simulink model "SW_8"  (R2013b)
settings: Solver=ode45  StartTime=0.0  StopTime=128  RelTol=1e-3
values from neighbouring files (symbols this model uses):
  const_val_lenqs = Nq-1    [confSim.m]    (also in preS_confSim.m)
  g = 1    [confSim.m]
  MiS = -5    [confSim.m]
  MS = 5    [confSim.m]
  nb_counter = ceil(log2(Ns))    [confSim.m]    (also in preS_confSim.m)
  NBitsScoreBus = 10    [confSim.m]    (also in preS_confSim.m)
  Nq = length(qCode)    [confSim.m]    (also in preS_confSim.m)
  Ns = length(sCode)    [confSim.m]    (also in preS_confSim.m)
  qCode = base2dec(q,Base)    [confSim.m]
  sCode = base2dec(s,Base)    [confSim.m]
  SMR_len = Nq*3    [confSim.m]    (also in preS_confSim.m)
libraries: xbsIndex_r4 x1212
(part 1 of 7)
settings Model: Creator=Fabio  LastModifiedBy=fabio

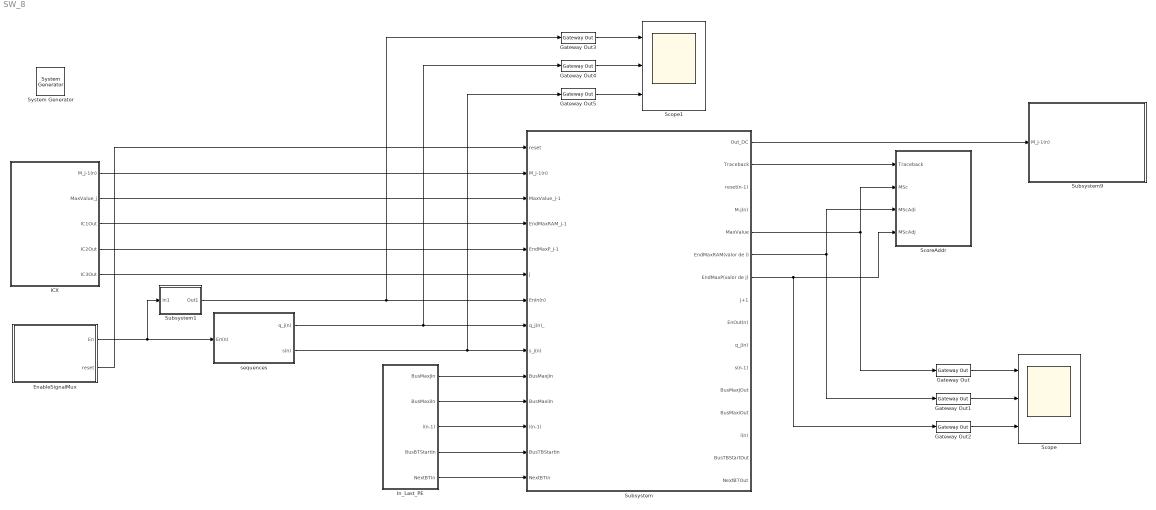
== system SW_8 ==
  " System Generator" : xbsIndex_r4/ System Generator  Tag=genX  xilinxfamily=virtex6  part=xc6vlx240t  speed=-1  package=ff1156  synthesis_tool=XST  clock_wrapper=Clock Enables  directory=./netlist  proj_type=Project Navigator  Synth_file=XST Defaults  Impl_file=ISE Defaults  testbench=off  simulink_period=Ts  sysclk_period=20  dcm_input_clock_period=10  incr_netlist=off  trim_vbits=Everywhere in SubSystem  dbl_ovrd=According to Block Masks  core_generation=According to Block Masks  run_coregen=off  deprecated_control=off  eval_field=0  block_type=sysgen
  "EnableSignalMux " : Subsystem
  Gateway Out{,1..5} (6 alike) : xbsIndex_r4/Gateway Out  inherit_from_input=off  hdl_port=on  timing_constraint=None  locs_specified=off  LOCs={}  UseAsDAC=off  DACChannel='1'  block_type=gatewayout
  ICX : Subsystem
  In_Last_PE : Subsystem
  Scope : Scope  NumInputPorts=3
      settings: YMin=-5~-5~-5  YMax=5~5~5
  Scope1 : Scope  NumInputPorts=3
      settings: YMin=-5~-5~-5  YMax=5~5~5
  ScoreAddr : Subsystem
  Subsystem : Subsystem
  Subsystem1 : Subsystem
  Subsystem9 : Subsystem
  sequences : Subsystem
  wires:
  ICX/1("M_j-1(n) ") -> Subsystem/2(M_j-1(n))
  ICX/2(MaxValue_j) -> Subsystem/3(MaxValue_j-1)
  ICX/3(IC1Out) -> Subsystem/4(EndMaxRAM_j-1)
  ICX/4(IC2Out) -> Subsystem/5(EndMaxP_j-1)
  ICX/5(IC3Out) -> Subsystem/6(j)
  "EnableSignalMux "/2(reset) -> Subsystem/1("reset ")
  In_Last_PE/1(BusMaxjIn) -> Subsystem/10(BusMaxjIn)
  In_Last_PE/2(BusMaxiIn) -> Subsystem/11(BusMaxiIn)
  In_Last_PE/3(i(n-1)) -> Subsystem/12(i(n-1))
  In_Last_PE/4(" BusBTStartIn") -> Subsystem/13(BusTBStartIn)
  In_Last_PE/5(NextBTIn) -> Subsystem/14(NextBTIn)
  Subsystem/1(Out_DC) -> Subsystem9/1(M_j-1(n))
  Subsystem/2(Traceback) -> ScoreAddr/1(Traceback)
  Subsystem/5(MaxValue) -> Gateway Out/1, ScoreAddr/2("MSc ")
  Subsystem/6(EndMaxRAM(valor de i)) -> Gateway Out1/1, ScoreAddr/3(MScAdi)
  Gateway Out/1 -> Scope/1
  Gateway Out1/1 -> Scope/2
  Gateway Out2/1 -> Scope/3
  Subsystem/7(EndMaxP(valor de j)) -> Gateway Out2/1, ScoreAddr/4(MScAdj)
  "EnableSignalMux "/1(En) -> Subsystem1/1(In1), sequences/1(En(n))
  sequences/1(q_j(n)) -> Subsystem/8(q_j(n)_), Gateway Out4/1
  Gateway Out3/1 -> Scope1/1
  Gateway Out4/1 -> Scope1/2
  Gateway Out5/1 -> Scope1/3
  sequences/2(s(n)) -> Gateway Out5/1, Subsystem/9(s_j(n))
  Subsystem1/1(Out1) -> Gateway Out3/1, Subsystem/7(EnIn(n))

== system SW_8/EnableSignalMux  ==
  Accumulator : xbsIndex_r4/Accumulator  operation=Add  n_bits=nbCR  overflow=Saturate  scale=1  rst=on  hasbypass=off  en=on  dbl_ovrd=off  use_behavioral_HDL=on  implementation=Fabric  block_type=accum
  Constant : xbsIndex_r4/Constant  const=1  gui_display_data_type=Fixed-point  arith_type=Unsigned  n_bits=1  bin_pt=0  preci_type=Single  exp_width=8  frac_width=24  explicit_period=on  period=tm  equ=P=C  opselect=C  inp2=PCIN>>17  opr=+  inp1=P  carry=CIN  dbl_ovrd=off  block_type=constant
  Constant1 : xbsIndex_r4/Constant  const=0  gui_display_data_type=Fixed-point  arith_type=Unsigned  n_bits=1  bin_pt=0  preci_type=Single  exp_width=8  frac_width=24  explicit_period=on  period=tm  equ=P=C  opselect=C  inp2=PCIN>>17  opr=+  inp1=P  carry=CIN  dbl_ovrd=off  block_type=constant
  Constant2 : xbsIndex_r4/Constant  const=Ns  gui_display_data_type=Fixed-point  arith_type=Unsigned  n_bits=nb_counter+1  bin_pt=0  preci_type=Single  exp_width=8  frac_width=24  explicit_period=on  period=tm  equ=P=C  opselect=C  inp2=PCIN>>17  opr=+  inp1=P  carry=CIN  dbl_ovrd=off  block_type=constant
  Convert2 : xbsIndex_r4/Convert  gui_display_data_type=Fixed-point  arith_type=Unsigned  n_bits=k  bin_pt=0  float_type=Single  exp_bits=8  fraction_bits=24  quantization=Truncate  overflow=Wrap  en=off  latency=c0  dbl_ovrd=off  pipeline=off  block_type=convert
  Convert5 : xbsIndex_r4/Convert  gui_display_data_type=Boolean  arith_type=Boolean  n_bits=4  bin_pt=0  float_type=Single  exp_bits=8  fraction_bits=24  quantization=Truncate  overflow=Wrap  en=off  latency=c0  dbl_ovrd=off  pipeline=off  block_type=convert
  From Register : xbsIndex_r4/From Register  shared_memory_name='En'  init=1  period=Ts  ownership=Locally owned and initialized  gui_display_data_type=Fixed-point  arith_type=Unsigned  n_bits=2  bin_pt=0  preci_type=Single  dbl_ovrd=off  block_type=fromreg
      settings: AttributesFormatString=<< %<shared_memory_name> >>  infoedit="Register block that reads data to a shared memory register.  Delay of one sample period."
  Inverter : xbsIndex_r4/Inverter  en=off  latency=l0  dbl_ovrd=off  block_type=inv
  Logical : xbsIndex_r4/Logical  logical_function=AND  inputs=2  en=off  latency=0  precision=Full  arith_type=Unsigned  n_bits=16  bin_pt=0  align_bp=on  dbl_ovrd=off  block_type=logical
  Mux : xbsIndex_r4/Mux  inputs=2  en=off  latency=0  precision=User Defined  arith_type=Unsigned  n_bits=nbEnMux  bin_pt=bpEnMux  quantization=Truncate  overflow=Wrap  dbl_ovrd=off  block_type=mux
  Relational : xbsIndex_r4/Relational  mode=a>=b  en=off  latency=r0  dbl_ovrd=off  block_type=relational
  Relational1 : xbsIndex_r4/Relational  mode=a>b  en=off  latency=r0  dbl_ovrd=off  block_type=relational
  "delay_reset " : xbsIndex_r4/Register  init=0  rst=off  en=off  dbl_ovrd=off  block_type=register
  En : Outport
  reset : Outport  Port=2
  wires:
  Constant/1 -> Mux/2
  Constant1/1 -> Relational1/2, Mux/3
  Constant2/1 -> Relational/2
  Accumulator/1 -> Relational/1
  Relational/1 -> Mux/1
  Mux/1 -> Convert5/1
  Convert5/1 -> Logical/2
  Logical/1 -> En/1
  Convert2/1 -> Accumulator/1
  From Register/1 -> Relational1/1
  Inverter/1 -> "delay_reset "/1, Accumulator/2
  "delay_reset "/1 -> reset/1
  Relational1/1 -> Accumulator/3, Logical/1, Convert2/1, Inverter/1

== system SW_8/ICX ==
  "ICM_j-1(n) " : xbsIndex_r4/Constant  const=0  gui_display_data_type=Fixed-point  arith_type=Signed (2's comp)  n_bits=NBitsIn  bin_pt=0  preci_type=Single  exp_width=8  frac_width=24  explicit_period=on  period=t0  equ=P=C  opselect=C  inp2=PCIN>>17  opr=+  inp1=P  carry=CIN  dbl_ovrd=off  block_type=constant
  ICMaxValue__j-1 : xbsIndex_r4/Constant  const=0  gui_display_data_type=Fixed-point  arith_type=Signed (2's comp)  n_bits=NBitsIn  bin_pt=0  preci_type=Single  exp_width=8  frac_width=24  explicit_period=on  period=t0  equ=P=C  opselect=C  inp2=PCIN>>17  opr=+  inp1=P  carry=CIN  dbl_ovrd=off  block_type=constant
  ICOut1 : xbsIndex_r4/Constant  const=0  gui_display_data_type=Fixed-point  arith_type=Signed (2's comp)  n_bits=NBitsIn  bin_pt=0  preci_type=Single  exp_width=8  frac_width=24  explicit_period=on  period=t0  equ=P=C  opselect=C  inp2=PCIN>>17  opr=+  inp1=P  carry=CIN  dbl_ovrd=off  block_type=constant
  ICOut2 : xbsIndex_r4/Constant  const=0  gui_display_data_type=Fixed-point  arith_type=Signed (2's comp)  n_bits=NBitsIn  bin_pt=0  preci_type=Single  exp_width=8  frac_width=24  explicit_period=on  period=t0  equ=P=C  opselect=C  inp2=PCIN>>17  opr=+  inp1=P  carry=CIN  dbl_ovrd=off  block_type=constant
  ICOut3 : xbsIndex_r4/Constant  const=0  gui_display_data_type=Fixed-point  arith_type=Signed (2's comp)  n_bits=NBitsIn  bin_pt=0  preci_type=Single  exp_width=8  frac_width=24  explicit_period=on  period=t0  equ=P=C  opselect=C  inp2=PCIN>>17  opr=+  inp1=P  carry=CIN  dbl_ovrd=off  block_type=constant
  "M_j-1(n) " : Outport
  MaxValue_j : Outport  Port=2
  IC1Out : Outport  Port=3
  IC2Out : Outport  Port=4
  IC3Out : Outport  Port=5
  wires:
  ICMaxValue__j-1/1 -> MaxValue_j/1
  "ICM_j-1(n) "/1 -> "M_j-1(n) "/1
  ICOut3/1 -> IC3Out/1
  ICOut2/1 -> IC2Out/1
  ICOut1/1 -> IC1Out/1

== system SW_8/In_Last_PE ==
  IC : xbsIndex_r4/Constant  const=0  gui_display_data_type=Fixed-point  arith_type=Unsigned  n_bits=3  bin_pt=0  preci_type=Single  exp_width=8  frac_width=24  explicit_period=on  period=Ts  equ=P=C  opselect=C  inp2=PCIN>>17  opr=+  inp1=P  carry=CIN  dbl_ovrd=off  block_type=constant
  IC1 : xbsIndex_r4/Constant  const=0  gui_display_data_type=Fixed-point  arith_type=Unsigned  n_bits=3  bin_pt=0  preci_type=Single  exp_width=8  frac_width=24  explicit_period=on  period=Ts  equ=P=C  opselect=C  inp2=PCIN>>17  opr=+  inp1=P  carry=CIN  dbl_ovrd=off  block_type=constant
  IC2 : xbsIndex_r4/Constant  const=0  gui_display_data_type=Fixed-point  arith_type=Unsigned  n_bits=NBitsIn  bin_pt=0  preci_type=Single  exp_width=8  frac_width=24  explicit_period=on  period=Ts  equ=P=C  opselect=C  inp2=PCIN>>17  opr=+  inp1=P  carry=CIN  dbl_ovrd=off  block_type=constant
  IC3 : xbsIndex_r4/Constant  const=0  gui_display_data_type=Fixed-point  arith_type=Unsigned  n_bits=1  bin_pt=0  preci_type=Single  exp_width=8  frac_width=24  explicit_period=on  period=Ts  equ=P=C  opselect=C  inp2=PCIN>>17  opr=+  inp1=P  carry=CIN  dbl_ovrd=off  block_type=constant
  IC5 : xbsIndex_r4/Constant  const=0  gui_display_data_type=Fixed-point  arith_type=Unsigned  n_bits=1  bin_pt=0  preci_type=Single  exp_width=8  frac_width=24  explicit_period=on  period=Ts  equ=P=C  opselect=C  inp2=PCIN>>17  opr=+  inp1=P  carry=CIN  dbl_ovrd=off  block_type=constant
  BusMaxjIn : Outport
  BusMaxiIn : Outport  Port=2
  i(n-1) : Outport  Port=3
  " BusBTStartIn" : Outport  Port=4
  NextBTIn : Outport  Port=5
  wires:
  IC3/1 -> " BusBTStartIn"/1
  IC1/1 -> BusMaxiIn/1
  IC5/1 -> NextBTIn/1
  IC2/1 -> i(n-1)/1
  IC/1 -> BusMaxjIn/1

== system SW_8/ScoreAddr ==
  Traceback : Inport
  "MSc " : Inport  Port=2
  MScAdi : Inport  Port=3
  MScAdj : Inport  Port=4
  Const_2 : xbsIndex_r4/Constant  const=2  gui_display_data_type=Fixed-point  arith_type=Unsigned  n_bits=k  bin_pt=kbp  preci_type=Single  exp_width=8  frac_width=24  explicit_period=off  period=1  equ=P=C  opselect=C  inp2=PCIN>>17  opr=+  inp1=P  carry=CIN  dbl_ovrd=off  block_type=constant
  Convert1 : xbsIndex_r4/Convert  gui_display_data_type=Boolean  arith_type=Boolean  n_bits=1  bin_pt=0  float_type=Single  exp_bits=8  fraction_bits=24  quantization=Truncate  overflow=Wrap  en=off  latency=c0  dbl_ovrd=off  pipeline=off  block_type=convert
  Counter : xbsIndex_r4/Counter  cnt_type=Count Limited  cnt_to=2  operation=Up  start_count=0  cnt_by_val=1  arith_type=Unsigned  n_bits=2  bin_pt=0  load_pin=off  rst=off  en=on  explicit_period=on  period=Ts  dbl_ovrd=off  use_behavioral_HDL=off  implementation=Fabric  block_type=counter
  Mux3 : xbsIndex_r4/Mux  inputs=3  en=off  latency=mft  precision=User Defined  arith_type=Unsigned  n_bits=NBitsCalcInt  bin_pt=0  quantization=Truncate  overflow=Wrap  dbl_ovrd=off  block_type=mux
  Register1 : xbsIndex_r4/Register  init=0  rst=on  en=on  dbl_ovrd=off  block_type=register
  Relational : xbsIndex_r4/Relational  mode=a=b  en=off  latency=0  dbl_ovrd=off  block_type=relational
  Shared Memory : xbsIndex_r4/Shared Memory  shared_memory_name='ScrnAddrs'  depth=3  ownership=Locally Owned and Initialized  initVector=zeros(1,3)  en=off  mutex=Unprotected  mode=Write Only  write_mode=No Read On Write  time_out=0  latency=Ts  explicit_data_type=on  gui_display_data_type=Fixed-point  arith_type=Unsigned  n_bits=16  bin_pt=0  preci_type=Single  implementation=Block RAM  use_rpm=off  block_type=shmem
      settings: AttributesFormatString=<< %<shared_memory_name> >>
  setEnable : Subsystem
  wires:
  Const_2/1 -> Relational/1
  Convert1/1 -> setEnable/1(In1), Register1/3, Register1/1
  Register1/1 -> Shared Memory/3
  Mux3/1 -> Shared Memory/2
  Counter/1 -> Relational/2, Shared Memory/1, Mux3/1
  "MSc "/1 -> Mux3/2
  MScAdi/1 -> Mux3/3
  setEnable/1(Out1) -> Counter/1
  Relational/1 -> Register1/2
  MScAdj/1 -> Mux3/4
  Traceback/1 -> Convert1/1

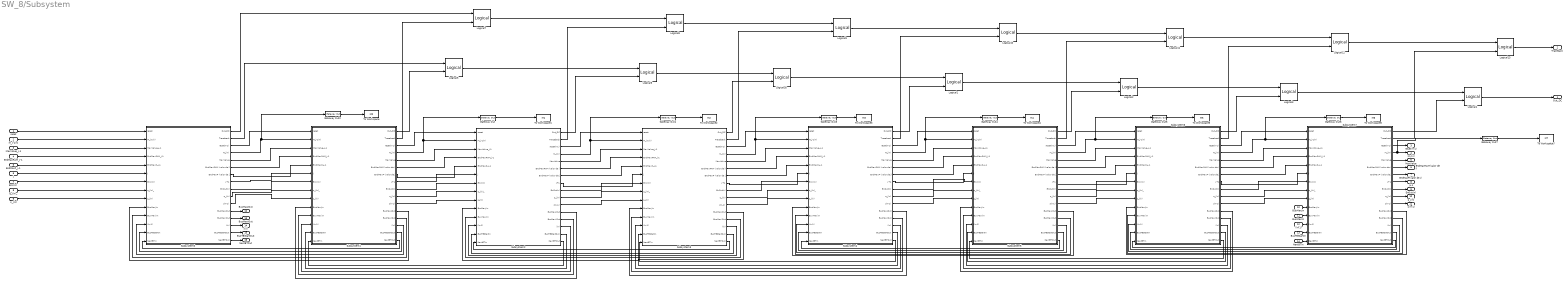
== system SW_8/Subsystem ==
  "reset " : Inport
  M_j-1(n) : Inport  Port=2
  MaxValue_j-1 : Inport  Port=3
  EndMaxRAM_j-1 : Inport  Port=4
  EndMaxP_j-1 : Inport  Port=5
  j : Inport  Port=6
  EnIn(n) : Inport  Port=7
  q_j(n)_ : Inport  Port=8
  s_j(n) : Inport  Port=9
  BusMaxjIn : Inport  Port=10
  BusMaxiIn : Inport  Port=11
  i(n-1) : Inport  Port=12
  BusTBStartIn : Inport  Port=13
  NextBTIn : Inport  Port=14
  Gateway Out{,1..7} (8 alike) : xbsIndex_r4/Gateway Out  inherit_from_input=off  hdl_port=on  timing_constraint=None  locs_specified=off  LOCs={}  UseAsDAC=off  DACChannel='1'  block_type=gatewayout
  Logical{1..6,35} (7 alike) : xbsIndex_r4/Logical  logical_function=XOR  inputs=2  en=off  latency=l0  precision=User Defined  arith_type=Unsigned  n_bits=k  bin_pt=0  align_bp=on  dbl_ovrd=off  block_type=logical
  Logical{7..13} (7 alike) : xbsIndex_r4/Logical  logical_function=XOR  inputs=2  en=off  latency=l0  precision=User Defined  arith_type=Unsigned  n_bits=nb_bool  bin_pt=0  align_bp=on  dbl_ovrd=off  block_type=logical
  Subsystem0 : Subsystem
  Subsystem1 : Subsystem
  Subsystem2 : Subsystem
  Subsystem3 : Subsystem
  Subsystem4 : Subsystem
  Subsystem5 : Subsystem
  Subsystem6 : Subsystem
  Subsystem7 : Subsystem
  To Workspace : ToWorkspace  VariableName=M0  SampleTime=-1
  To Workspace1 : ToWorkspace  VariableName=M1  SampleTime=-1
  To Workspace2 : ToWorkspace  VariableName=M2  SampleTime=-1
  To Workspace3 : ToWorkspace  VariableName=M3  SampleTime=-1
  To Workspace4 : ToWorkspace  VariableName=M4  SampleTime=-1
  To Workspace5 : ToWorkspace  VariableName=M5  SampleTime=-1
  To Workspace6 : ToWorkspace  VariableName=M6  SampleTime=-1
  To Workspace7 : ToWorkspace  VariableName=M7  SampleTime=-1
  Out_DC : Outport
  Traceback : Outport  Port=2
  reset(n-1) : Outport  Port=3
  M-j(n) : Outport  Port=4
  MaxValue : Outport  Port=5
  EndMaxRAM(valor de i) : Outport  Port=6
  EndMaxP(valor de j) : Outport  Port=7
  j+1 : Outport  Port=8
  EnOut(n) : Outport  Port=9
  q_j(n) : Outport  Port=10
  s(n-1) : Outport  Port=11
  BusMaxjOut : Outport  Port=12
  BusMaxiOut : Outport  Port=13
  i(n) : Outport  Port=14
  BusTBStartOut : Outport  Port=15
  NextBTOut : Outport  Port=16
  wires:
  Subsystem4/1("Out_DC ") -> Logical1/2
  s_j(n)/1 -> Subsystem0/9(s_j(n))
  M_j-1(n)/1 -> Subsystem0/2(M_j-1(n))
  j/1 -> Subsystem0/6(j)
  EndMaxRAM_j-1/1 -> Subsystem0/4(EndMaxRAM_j-1)
  MaxValue_j-1/1 -> Subsystem0/3(MaxValue_j-1)
  q_j(n)_/1 -> Subsystem0/8(q_j(n)_)
  EndMaxP_j-1/1 -> Subsystem0/5(EndMaxP_j-1)
  EnIn(n)/1 -> Subsystem0/7(EnIn(n))
  BusTBStartIn/1 -> Subsystem7/13(BusTBStartIn)
  NextBTIn/1 -> Subsystem7/14(NextBTIn)
  Subsystem7/5(MaxValue) -> MaxValue/1
  Subsystem7/6(EndMaxRAM (valor de i)) -> EndMaxRAM(valor de i)/1
  Subsystem7/7(EndMaxP (valor de j)) -> EndMaxP(valor de j)/1
  Subsystem7/8(j+1) -> j+1/1
  Subsystem7/9(EnOut(n)) -> EnOut(n)/1
  Subsystem7/10(q_j(n)) -> q_j(n)/1
  Subsystem7/11(s(n-1)) -> s(n-1)/1
  Logical35/1 -> Logical1/1
  Logical1/1 -> Logical2/1
  Subsystem3/1("Out_DC ") -> Logical35/2
  Subsystem7/1("Out_DC ") -> Logical4/2
  Logical2/1 -> Logical3/1
  Logical3/1 -> Logical4/1
  Subsystem6/1("Out_DC ") -> Logical3/2
  Subsystem5/2(Traceback) -> Logical11/2
  Subsystem5/1("Out_DC ") -> Logical2/2
  Logical9/1 -> Logical10/1
  Logical4/1 -> Out_DC/1
  Subsystem0/12(BusMaxjOut) -> BusMaxjOut/1
  Logical13/1 -> Traceback/1
  Subsystem0/13(BusMaxiOut) -> BusMaxiOut/1
  Subsystem0/16(NextBTOut) -> NextBTOut/1
  BusMaxiIn/1 -> Subsystem7/11(BuxMaxiIn)
  i(n-1)/1 -> Subsystem7/12(i(n-1))
  Subsystem0/15(BusTBStartOut) -> BusTBStartOut/1
  BusMaxjIn/1 -> Subsystem7/10(BusMaxjIn)
  Subsystem0/14(i(n)) -> i(n)/1
  Subsystem1/1("Out_DC ") -> Logical5/2
  Logical12/1 -> Logical13/1
  Subsystem2/2(Traceback) -> Logical8/2
  Logical7/1 -> Logical8/1
  Subsystem7/2(Traceback) -> Logical13/2
  Logical11/1 -> Logical12/1
  Logical8/1 -> Logical9/1
  Logical10/1 -> Logical11/1
  Logical6/1 -> Logical35/1
  Subsystem6/2(Traceback) -> Logical12/2
  Subsystem3/2(Traceback) -> Logical9/2
  Logical5/1 -> Logical6/1
  Subsystem2/1("Out_DC ") -> Logical6/2
  Subsystem4/2(Traceback) -> Logical10/2
  "reset "/1 -> Subsystem0/1("reset ")
  Subsystem0/3(reset(n-1)) -> Subsystem1/1("reset ")
  Subsystem0/5(MaxValue) -> Subsystem1/3(MaxValue_j-1)
  Subsystem0/6(EndMaxRAM (valor de i)) -> Subsystem1/4(EndMaxRAM_j-1)
  Subsystem0/7(EndMaxP (valor de j)) -> Subsystem1/5(EndMaxP_j-1)
  Subsystem0/8(j+1) -> Subsystem1/6(j)
  Subsystem0/9(EnOut(n)) -> Subsystem1/7(EnIn(n))
  Subsystem0/10(q_j(n)) -> Subsystem1/8(q_j(n)_)
  Subsystem0/11(s(n-1)) -> Subsystem1/9(s_j(n))
  Subsystem1/3(reset(n-1)) -> Subsystem2/1("reset ")
  Subsystem1/5(MaxValue) -> Subsystem2/3(MaxValue_j-1)
  Subsystem1/6(EndMaxRAM (valor de i)) -> Subsystem2/4(EndMaxRAM_j-1)
  Subsystem1/7(EndMaxP (valor de j)) -> Subsystem2/5(EndMaxP_j-1)
  Subsystem1/8(j+1) -> Subsystem2/6(j)
  Subsystem1/9(EnOut(n)) -> Subsystem2/7(EnIn(n))
  Subsystem1/10(q_j(n)) -> Subsystem2/8(q_j(n)_)
  Subsystem1/11(s(n-1)) -> Subsystem2/9(s_j(n))
  Subsystem2/3(reset(n-1)) -> Subsystem3/1("reset ")
  Subsystem2/5(MaxValue) -> Subsystem3/3(MaxValue_j-1)
  Subsystem2/6(EndMaxRAM (valor de i)) -> Subsystem3/4(EndMaxRAM_j-1)
  Subsystem2/7(EndMaxP (valor de j)) -> Subsystem3/5(EndMaxP_j-1)
  Subsystem2/8(j+1) -> Subsystem3/6(j)
  Subsystem2/9(EnOut(n)) -> Subsystem3/7(EnIn(n))
  Subsystem2/10(q_j(n)) -> Subsystem3/8(q_j(n)_)
  Subsystem2/11(s(n-1)) -> Subsystem3/9(s_j(n))
  Subsystem3/3(reset(n-1)) -> Subsystem4/1("reset ")
  Subsystem3/5(MaxValue) -> Subsystem4/3(MaxValue_j-1)
  Subsystem3/6(EndMaxRAM (valor de i)) -> Subsystem4/4(EndMaxRAM_j-1)
  Subsystem3/7(EndMaxP (valor de j)) -> Subsystem4/5(EndMaxP_j-1)
  Subsystem3/8(j+1) -> Subsystem4/6(j)
  Subsystem3/9(EnOut(n)) -> Subsystem4/7(EnIn(n))
  Subsystem3/10(q_j(n)) -> Subsystem4/8(q_j(n)_)
  Subsystem3/11(s(n-1)) -> Subsystem4/9(s_j(n))
  Subsystem4/3(reset(n-1)) -> Subsystem5/1("reset ")
  Subsystem4/5(MaxValue) -> Subsystem5/3(MaxValue_j-1)
  Subsystem4/6(EndMaxRAM (valor de i)) -> Subsystem5/4(EndMaxRAM_j-1)
  Subsystem4/7(EndMaxP (valor de j)) -> Subsystem5/5(EndMaxP_j-1)
  Subsystem4/8(j+1) -> Subsystem5/6(j)
  Subsystem4/9(EnOut(n)) -> Subsystem5/7(EnIn(n))
  Subsystem4/10(q_j(n)) -> Subsystem5/8(q_j(n)_)
  Subsystem4/11(s(n-1)) -> Subsystem5/9(s_j(n))
  Subsystem5/3(reset(n-1)) -> Subsystem6/1("reset ")
  Subsystem5/5(MaxValue) -> Subsystem6/3(MaxValue_j-1)
  Subsystem5/6(EndMaxRAM (valor de i)) -> Subsystem6/4(EndMaxRAM_j-1)
  Subsystem5/7(EndMaxP (valor de j)) -> Subsystem6/5(EndMaxP_j-1)
  Subsystem5/8(j+1) -> Subsystem6/6(j)
  Subsystem5/9(EnOut(n)) -> Subsystem6/7(EnIn(n))
  Subsystem5/10(q_j(n)) -> Subsystem6/8(q_j(n)_)
  Subsystem5/11(s(n-1)) -> Subsystem6/9(s_j(n))
  Subsystem6/3(reset(n-1)) -> Subsystem7/1("reset ")
  Subsystem6/5(MaxValue) -> Subsystem7/3(MaxValue_j-1)
  Subsystem6/6(EndMaxRAM (valor de i)) -> Subsystem7/4(EndMaxRAM_j-1)
  Subsystem6/7(EndMaxP (valor de j)) -> Subsystem7/5(EndMaxP_j-1)
  Subsystem6/8(j+1) -> Subsystem7/6(j)
  Subsystem6/9(EnOut(n)) -> Subsystem7/7(EnIn(n))
  Subsystem6/10(q_j(n)) -> Subsystem7/8(q_j(n)_)
  Subsystem6/11(s(n-1)) -> Subsystem7/9(s_j(n))
  Subsystem7/3(reset(n-1)) -> reset(n-1)/1
  Subsystem1/2(Traceback) -> Logical7/2
  Subsystem7/16(NextBTOut) -> Subsystem6/14(NextBTIn)
  Subsystem7/15(BusTBStartOut) -> Subsystem6/13(BusTBStartIn)
  Subsystem7/14(i(n)) -> Subsystem6/12(i(n-1))
  Subsystem3/16(NextBTOut) -> Subsystem2/14(NextBTIn)
  Subsystem7/13(BusMaxiOut) -> Subsystem6/11(BuxMaxiIn)
  Subsystem7/12(BusMaxjOut) -> Subsystem6/10(BusMaxjIn)
  Subsystem6/16(NextBTOut) -> Subsystem5/14(NextBTIn)
  Subsystem6/15(BusTBStartOut) -> Subsystem5/13(BusTBStartIn)
  Subsystem6/14(i(n)) -> Subsystem5/12(i(n-1))
  Subsystem6/13(BusMaxiOut) -> Subsystem5/11(BuxMaxiIn)
  Subsystem6/12(BusMaxjOut) -> Subsystem5/10(BusMaxjIn)
  Subsystem5/16(NextBTOut) -> Subsystem4/14(NextBTIn)
  Subsystem5/15(BusTBStartOut) -> Subsystem4/13(BusTBStartIn)
  Subsystem5/14(i(n)) -> Subsystem4/12(i(n-1))
  Subsystem5/13(BusMaxiOut) -> Subsystem4/11(BuxMaxiIn)
  Subsystem5/12(BusMaxjOut) -> Subsystem4/10(BusMaxjIn)
  Subsystem4/16(NextBTOut) -> Subsystem3/14(NextBTIn)
  Subsystem4/15(BusTBStartOut) -> Subsystem3/13(BusTBStartIn)
  Subsystem4/14(i(n)) -> Subsystem3/12(i(n-1))
  Subsystem4/13(BusMaxiOut) -> Subsystem3/11(BuxMaxiIn)
  Subsystem4/12(BusMaxjOut) -> Subsystem3/10(BusMaxjIn)
  Subsystem3/15(BusTBStartOut) -> Subsystem2/13(BusTBStartIn)
  Subsystem3/14(i(n)) -> Subsystem2/12(i(n-1))
  Subsystem3/13(BusMaxiOut) -> Subsystem2/11(BuxMaxiIn)
  Subsystem3/12(BusMaxjOut) -> Subsystem2/10(BusMaxjIn)
  Subsystem2/16(NextBTOut) -> Subsystem1/14(NextBTIn)
  Subsystem2/15(BusTBStartOut) -> Subsystem1/13(BusTBStartIn)
  Subsystem2/14(i(n)) -> Subsystem1/12(i(n-1))
  Subsystem2/13(BusMaxiOut) -> Subsystem1/11(BuxMaxiIn)
  Subsystem2/12(BusMaxjOut) -> Subsystem1/10(BusMaxjIn)
  Subsystem1/16(NextBTOut) -> Subsystem0/14(NextBTIn)
  Subsystem1/15(BusTBStartOut) -> Subsystem0/13(BusTBStartIn)
  Subsystem1/14(i(n)) -> Subsystem0/12(i(n-1))
  Subsystem1/13(BusMaxiOut) -> Subsystem0/11(BuxMaxiIn)
  Subsystem1/12(BusMaxjOut) -> Subsystem0/10(BusMaxjIn)
  Subsystem0/4(M_j(n)) -> Gateway Out2/1, Subsystem1/2(M_j-1(n))
  Subsystem1/4(M_j(n)) -> Gateway Out/1, Subsystem2/2(M_j-1(n))
  Subsystem2/4(M_j(n)) -> Gateway Out1/1, Subsystem3/2(M_j-1(n))
  Subsystem3/4(M_j(n)) -> Gateway Out3/1, Subsystem4/2(M_j-1(n))
  Subsystem4/4(M_j(n)) -> Gateway Out4/1, Subsystem5/2(M_j-1(n))
  Subsystem5/4(M_j(n)) -> Gateway Out5/1, Subsystem6/2(M_j-1(n))
  Subsystem6/4(M_j(n)) -> Gateway Out6/1, Subsystem7/2(M_j-1(n))
  Subsystem7/4(M_j(n)) -> Gateway Out7/1, M-j(n)/1
  Gateway Out/1 -> To Workspace1/1
  Gateway Out1/1 -> To Workspace2/1
  Gateway Out2/1 -> To Workspace/1
  Gateway Out3/1 -> To Workspace3/1
  Gateway Out4/1 -> To Workspace4/1
  Gateway Out5/1 -> To Workspace5/1
  Gateway Out6/1 -> To Workspace6/1
  Gateway Out7/1 -> To Workspace7/1
  Subsystem0/1("Out_DC ") -> Logical7/1
  Subsystem0/2(Traceback) -> Logical5/1

== system SW_8/Subsystem1 ==
  In1 : Inport
  Register1 : xbsIndex_r4/Register  init=0  rst=off  en=off  dbl_ovrd=off  block_type=register
  Register2 : xbsIndex_r4/Register  init=0  rst=off  en=off  dbl_ovrd=off  block_type=register
  Out1 : Outport
  wires:
  In1/1 -> Register2/1
  Register1/1 -> Out1/1
  Register2/1 -> Register1/1

== system SW_8/Subsystem9 ==
  M_j-1(n) : Inport
  Accumulator : xbsIndex_r4/Accumulator  operation=Add  n_bits=nb_SMR  overflow=Saturate  scale=1  rst=off  hasbypass=off  en=off  dbl_ovrd=off  use_behavioral_HDL=on  implementation=Fabric  block_type=accum
  Const_2 : xbsIndex_r4/Constant  const=0  gui_display_data_type=Fixed-point  arith_type=Unsigned  n_bits=counter_num_b  bin_pt=kbp  preci_type=Single  exp_width=8  frac_width=24  explicit_period=off  period=1  equ=P=C  opselect=C  inp2=PCIN>>17  opr=+  inp1=P  carry=CIN  dbl_ovrd=off  block_type=constant
  Convert1 : xbsIndex_r4/Convert  gui_display_data_type=Boolean  arith_type=Boolean  n_bits=1  bin_pt=0  float_type=Single  exp_bits=8  fraction_bits=24  quantization=Truncate  overflow=Wrap  en=off  latency=c0  dbl_ovrd=off  pipeline=off  block_type=convert
  Convert2 : xbsIndex_r4/Convert  gui_display_data_type=Fixed-point  arith_type=Unsigned  n_bits=nb_bool  bin_pt=0  float_type=Single  exp_bits=8  fraction_bits=24  quantization=Truncate  overflow=Wrap  en=off  latency=c0  dbl_ovrd=off  pipeline=off  block_type=convert
  Register : xbsIndex_r4/Register  init=0  rst=off  en=off  dbl_ovrd=off  block_type=register
  Register1 : xbsIndex_r4/Register  init=0  rst=off  en=off  dbl_ovrd=off  block_type=register
  Register2 : xbsIndex_r4/Register  init=0  rst=off  en=off  dbl_ovrd=off  block_type=register
  Relational : xbsIndex_r4/Relational  mode=a<b  en=off  latency=r0  dbl_ovrd=off  block_type=relational
  Shared Memory : xbsIndex_r4/Shared Memory  shared_memory_name='SMR2'  depth=SMR_len  ownership=Locally Owned and Initialized  initVector=zeros(1,SMR_len)  en=off  mutex=Unprotected  mode=Write Only  write_mode=No Read On Write  time_out=0  latency=Ts  explicit_data_type=on  gui_display_data_type=Fixed-point  arith_type=Unsigned  n_bits=k  bin_pt=kbp  preci_type=Single  implementation=Block RAM  use_rpm=off  block_type=shmem
      settings: AttributesFormatString=<< %<shared_memory_name> >>
  wires:
  Register/1 -> Shared Memory/2
  Convert2/1 -> Convert1/1, Accumulator/1
  Relational/1 -> Convert2/1
  Register2/1 -> Shared Memory/1
  Convert1/1 -> Register1/1
  Const_2/1 -> Relational/1
  Accumulator/1 -> Register2/1
  Register1/1 -> Shared Memory/3
  M_j-1(n)/1 -> Relational/2, Register/1

== system SW_8/sequences ==
  En(n) : Inport
  Convert : xbsIndex_r4/Convert  gui_display_data_type=Fixed-point  arith_type=Unsigned  n_bits=nb_bool  bin_pt=bp_bool  float_type=Single  exp_bits=8  fraction_bits=24  quantization=Truncate  overflow=Wrap  en=off  latency=0  dbl_ovrd=off  pipeline=off  block_type=convert
  "qCode " : Subsystem
  sCode : Subsystem
  q_j(n) : Outport
  s(n) : Outport  Port=2
  wires:
  "qCode "/1(qc) -> q_j(n)/1
  sCode/1(sc) -> s(n)/1
  En(n)/1 -> Convert/1
  Convert/1 -> sCode/1(EnS), "qCode "/1("EnQ ")

== system SW_8/ScoreAddr/setEnable ==
  In1 : Inport
  Register1 : xbsIndex_r4/Register  init=0  rst=off  en=on  dbl_ovrd=off  block_type=register
  Out1 : Outport
  wires:
  Register1/1 -> Out1/1
  In1/1 -> Register1/2, Register1/1

== system SW_8/Subsystem/Subsystem0 ==
  "reset " : Inport
  M_j-1(n) : Inport  Port=2
  MaxValue_j-1 : Inport  Port=3
  EndMaxRAM_j-1 : Inport  Port=4
  EndMaxP_j-1 : Inport  Port=5
  j : Inport  Port=6
  EnIn(n) : Inport  Port=7
  q_j(n)_ : Inport  Port=8
  s_j(n) : Inport  Port=9
  BusMaxjIn : Inport  Port=10
  BuxMaxiIn : Inport  Port=11
  i(n-1) : Inport  Port=12
  BusTBStartIn : Inport  Port=13
  NextBTIn : Inport  Port=14
  Backtracking_final : Subsystem
  P1_HW0 : Subsystem
  Register1 : xbsIndex_r4/Register  init=0  rst=off  en=off  dbl_ovrd=off  block_type=register
  Register10 : xbsIndex_r4/Register  init=0  rst=off  en=off  dbl_ovrd=off  block_type=register
  _RAM_0 : Subsystem
  "delay_reset " : xbsIndex_r4/Register  init=0  rst=off  en=off  dbl_ovrd=off  block_type=register
  delay_tc{,1..7} (8 alike) : xbsIndex_r4/Register  init=0  rst=off  en=off  dbl_ovrd=off  block_type=register
  seq_switch : Subsystem
  "Out_DC " : Outport
  Traceback : Outport  Port=2
  reset(n-1) : Outport  Port=3
  M_j(n) : Outport  Port=4
  MaxValue : Outport  Port=5
  EndMaxRAM (valor de i) : Outport  Port=6
  EndMaxP (valor de j) : Outport  Port=7
  j+1 : Outport  Port=8
  EnOut(n) : Outport  Port=9
  q_j(n) : Outport  Port=10
  s(n-1) : Outport  Port=11
  BusMaxjOut : Outport  Port=12
  BusMaxiOut : Outport  Port=13
  i(n) : Outport  Port=14
  BusTBStartOut : Outport  Port=15
  NextBTOut : Outport  Port=16
  wires:
  Backtracking_final/3(Out_DC_j(n)) -> Register10/1
  _RAM_0/1(D_j(n)1) -> Backtracking_final/2("D(j)_n ")
  delay_tc7/1 -> BusMaxjOut/1
  delay_tc6/1 -> NextBTOut/1
  delay_tc5/1 -> i(n)/1
  delay_tc4/1 -> BusTBStartOut/1
  delay_tc3/1 -> BusMaxiOut/1
  delay_tc/1 -> MaxValue/1
  delay_tc2/1 -> EndMaxP (valor de j)/1
  delay_tc1/1 -> EndMaxRAM (valor de i)/1
  EndMaxRAM_j-1/1 -> P1_HW0/4(EndMaxRAM_j-1)
  M_j-1(n)/1 -> P1_HW0/2(M_j-1(n)1)
  j/1 -> P1_HW0/6(j-1)
  seq_switch/1(q_j) -> P1_HW0/9(q_j)
  MaxValue_j-1/1 -> P1_HW0/3(MaxValue_j-1)
  EndMaxP_j-1/1 -> P1_HW0/5(EndMaxP_j-1)
  EnIn(n)/1 -> P1_HW0/8(EnIn), _RAM_0/1(En(n)), seq_switch/2("Enable ")
  Backtracking_final/6(BusTBStartOut) -> delay_tc4/1
  Backtracking_final/8(NextBTOut) -> delay_tc6/1
  BusMaxjIn/1 -> Backtracking_final/7(BusMaxjIn)
  BusTBStartIn/1 -> Backtracking_final/9(BusTBStartIn)
  NextBTIn/1 -> Backtracking_final/11(NextBTIn)
  P1_HW0/11(out_j) -> Backtracking_final/6(j)
  P1_HW0/3(EndMaxRAM (valor de i)) -> Backtracking_final/5(Maxi), delay_tc1/1
  Backtracking_final/1(BT_RAM_j(n)=i) -> _RAM_0/4(BT_RAM_j(n)=i)
  i(n-1)/1 -> Backtracking_final/10(i(n-1))
  Backtracking_final/4(BusMaxjOut) -> delay_tc7/1
  Backtracking_final/5(BusMaxiOut) -> delay_tc3/1
  BuxMaxiIn/1 -> Backtracking_final/8(BusMaxiIn)
  Backtracking_final/7(i(n)) -> delay_tc5/1
  Backtracking_final/2(BTRAMCont) -> _RAM_0/5(BTRAMCont)
  P1_HW0/4(EndMaxP (valor de j)) -> Backtracking_final/4(Maxj), delay_tc2/1
  P1_HW0/1(M_j(n)) -> M_j(n)/1
  P1_HW0/2(MaxValue) -> delay_tc/1
  P1_HW0/9(wEnd) -> _RAM_0/2(RAM_j(n)=i)
  P1_HW0/8(Direction) -> _RAM_0/3(D_j(n))
  P1_HW0/6(s(n-1)) -> s(n-1)/1
  P1_HW0/5(j) -> j+1/1
  P1_HW0/7(EnOut(n)) -> EnOut(n)/1
  seq_switch/2(q_j(n-1)) -> q_j(n)/1
  q_j(n)_/1 -> seq_switch/1(q_j(n))
  s_j(n)/1 -> P1_HW0/7(s(n))
  P1_HW0/10(TraceBackStart) -> Backtracking_final/3(TraceBackStart), Register1/1
  "reset "/1 -> P1_HW0/1("reset "), Backtracking_final/1("reset "), "delay_reset "/1, seq_switch/3("reset ")
  "delay_reset "/1 -> reset(n-1)/1
  Register10/1 -> "Out_DC "/1
  Register1/1 -> Traceback/1

== system SW_8/Subsystem/Subsystem1 ==
  "reset " : Inport
  M_j-1(n) : Inport  Port=2
  MaxValue_j-1 : Inport  Port=3
  EndMaxRAM_j-1 : Inport  Port=4
  EndMaxP_j-1 : Inport  Port=5
  j : Inport  Port=6
  EnIn(n) : Inport  Port=7
  q_j(n)_ : Inport  Port=8
  s_j(n) : Inport  Port=9
  BusMaxjIn : Inport  Port=10
  BuxMaxiIn : Inport  Port=11
  i(n-1) : Inport  Port=12
  BusTBStartIn : Inport  Port=13
  NextBTIn : Inport  Port=14
  Backtracking_final : Subsystem
  P1_HW0 : Subsystem
  Register1 : xbsIndex_r4/Register  init=0  rst=off  en=off  dbl_ovrd=off  block_type=register
  Register10 : xbsIndex_r4/Register  init=0  rst=off  en=off  dbl_ovrd=off  block_type=register
  _RAM_0 : Subsystem
  "delay_reset " : xbsIndex_r4/Register  init=0  rst=off  en=off  dbl_ovrd=off  block_type=register
  delay_tc{,1..7} (8 alike) : xbsIndex_r4/Register  init=0  rst=off  en=off  dbl_ovrd=off  block_type=register
  seq_switch : Subsystem
  "Out_DC " : Outport
  Traceback : Outport  Port=2
  reset(n-1) : Outport  Port=3
  M_j(n) : Outport  Port=4
  MaxValue : Outport  Port=5
  EndMaxRAM (valor de i) : Outport  Port=6
  EndMaxP (valor de j) : Outport  Port=7
  j+1 : Outport  Port=8
  EnOut(n) : Outport  Port=9
  q_j(n) : Outport  Port=10
  s(n-1) : Outport  Port=11
  BusMaxjOut : Outport  Port=12
  BusMaxiOut : Outport  Port=13
  i(n) : Outport  Port=14
  BusTBStartOut : Outport  Port=15
  NextBTOut : Outport  Port=16
  wires:
  Backtracking_final/3(Out_DC_j(n)) -> Register10/1
  _RAM_0/1(D_j(n)1) -> Backtracking_final/2("D(j)_n ")
  delay_tc7/1 -> BusMaxjOut/1
  delay_tc6/1 -> NextBTOut/1
  delay_tc5/1 -> i(n)/1
  delay_tc4/1 -> BusTBStartOut/1
  delay_tc3/1 -> BusMaxiOut/1
  delay_tc/1 -> MaxValue/1
  delay_tc2/1 -> EndMaxP (valor de j)/1
  delay_tc1/1 -> EndMaxRAM (valor de i)/1
  EndMaxRAM_j-1/1 -> P1_HW0/4(EndMaxRAM_j-1)
  M_j-1(n)/1 -> P1_HW0/2(M_j-1(n)1)
  j/1 -> P1_HW0/6(j-1)
  seq_switch/1(q_j) -> P1_HW0/9(q_j)
  MaxValue_j-1/1 -> P1_HW0/3(MaxValue_j-1)
  EndMaxP_j-1/1 -> P1_HW0/5(EndMaxP_j-1)
  EnIn(n)/1 -> P1_HW0/8(EnIn), seq_switch/2("Enable "), _RAM_0/1(En(n))
  Backtracking_final/6(BusTBStartOut) -> delay_tc4/1
  Backtracking_final/8(NextBTOut) -> delay_tc6/1
  BusMaxjIn/1 -> Backtracking_final/7(BusMaxjIn)
  BusTBStartIn/1 -> Backtracking_final/9(BusTBStartIn)
  NextBTIn/1 -> Backtracking_final/11(NextBTIn)
  P1_HW0/11(out_j) -> Backtracking_final/6(j)
  P1_HW0/3(EndMaxRAM (valor de i)) -> Backtracking_final/5(Maxi), delay_tc1/1
  Backtracking_final/1(BT_RAM_j(n)=i) -> _RAM_0/4(BT_RAM_j(n)=i)
  i(n-1)/1 -> Backtracking_final/10(i(n-1))
  Backtracking_final/4(BusMaxjOut) -> delay_tc7/1
  Backtracking_final/5(BusMaxiOut) -> delay_tc3/1
  BuxMaxiIn/1 -> Backtracking_final/8(BusMaxiIn)
  Backtracking_final/7(i(n)) -> delay_tc5/1
  Backtracking_final/2(BTRAMCont) -> _RAM_0/5(BTRAMCont)
  P1_HW0/4(EndMaxP (valor de j)) -> Backtracking_final/4(Maxj), delay_tc2/1
  P1_HW0/1(M_j(n)) -> M_j(n)/1
  P1_HW0/2(MaxValue) -> delay_tc/1
  P1_HW0/9(wEnd) -> _RAM_0/2(RAM_j(n)=i)
  P1_HW0/8(Direction) -> _RAM_0/3(D_j(n))
  P1_HW0/6(s(n-1)) -> s(n-1)/1
  P1_HW0/5(j) -> j+1/1
  P1_HW0/7(EnOut(n)) -> EnOut(n)/1
  seq_switch/2(q_j(n-1)) -> q_j(n)/1
  q_j(n)_/1 -> seq_switch/1(q_j(n))
  s_j(n)/1 -> P1_HW0/7(s(n))
  P1_HW0/10(TraceBackStart) -> Backtracking_final/3(TraceBackStart), Register1/1
  "reset "/1 -> P1_HW0/1("reset "), Backtracking_final/1("reset "), "delay_reset "/1, seq_switch/3("reset ")
  "delay_reset "/1 -> reset(n-1)/1
  Register10/1 -> "Out_DC "/1
  Register1/1 -> Traceback/1

== system SW_8/Subsystem/Subsystem2 ==
  "reset " : Inport
  M_j-1(n) : Inport  Port=2
  MaxValue_j-1 : Inport  Port=3
  EndMaxRAM_j-1 : Inport  Port=4
  EndMaxP_j-1 : Inport  Port=5
  j : Inport  Port=6
  EnIn(n) : Inport  Port=7
  q_j(n)_ : Inport  Port=8
  s_j(n) : Inport  Port=9
  BusMaxjIn : Inport  Port=10
  BuxMaxiIn : Inport  Port=11
  i(n-1) : Inport  Port=12
  BusTBStartIn : Inport  Port=13
  NextBTIn : Inport  Port=14
  Backtracking_final : Subsystem
  P1_HW0 : Subsystem
  Register1 : xbsIndex_r4/Register  init=0  rst=off  en=off  dbl_ovrd=off  block_type=register
  Register10 : xbsIndex_r4/Register  init=0  rst=off  en=off  dbl_ovrd=off  block_type=register
  _RAM_0 : Subsystem
  "delay_reset " : xbsIndex_r4/Register  init=0  rst=off  en=off  dbl_ovrd=off  block_type=register
  delay_tc{,1..7} (8 alike) : xbsIndex_r4/Register  init=0  rst=off  en=off  dbl_ovrd=off  block_type=register
  seq_switch : Subsystem
  "Out_DC " : Outport
  Traceback : Outport  Port=2
  reset(n-1) : Outport  Port=3
  M_j(n) : Outport  Port=4
  MaxValue : Outport  Port=5
  EndMaxRAM (valor de i) : Outport  Port=6
  EndMaxP (valor de j) : Outport  Port=7
  j+1 : Outport  Port=8
  EnOut(n) : Outport  Port=9
  q_j(n) : Outport  Port=10
  s(n-1) : Outport  Port=11
  BusMaxjOut : Outport  Port=12
  BusMaxiOut : Outport  Port=13
  i(n) : Outport  Port=14
  BusTBStartOut : Outport  Port=15
  NextBTOut : Outport  Port=16
  wires:
  Backtracking_final/3(Out_DC_j(n)) -> Register10/1
  _RAM_0/1(D_j(n)1) -> Backtracking_final/2("D(j)_n ")
  delay_tc7/1 -> BusMaxjOut/1
  delay_tc6/1 -> NextBTOut/1
  delay_tc5/1 -> i(n)/1
  delay_tc4/1 -> BusTBStartOut/1
  delay_tc3/1 -> BusMaxiOut/1
  delay_tc/1 -> MaxValue/1
  delay_tc2/1 -> EndMaxP (valor de j)/1
  delay_tc1/1 -> EndMaxRAM (valor de i)/1
  EndMaxRAM_j-1/1 -> P1_HW0/4(EndMaxRAM_j-1)
  M_j-1(n)/1 -> P1_HW0/2(M_j-1(n)1)
  j/1 -> P1_HW0/6(j-1)
  seq_switch/1(q_j) -> P1_HW0/9(q_j)
  MaxValue_j-1/1 -> P1_HW0/3(MaxValue_j-1)
  EndMaxP_j-1/1 -> P1_HW0/5(EndMaxP_j-1)
  EnIn(n)/1 -> P1_HW0/8(EnIn), seq_switch/2("Enable "), _RAM_0/1(En(n))
  Backtracking_final/6(BusTBStartOut) -> delay_tc4/1
  Backtracking_final/8(NextBTOut) -> delay_tc6/1
  BusMaxjIn/1 -> Backtracking_final/7(BusMaxjIn)
  BusTBStartIn/1 -> Backtracking_final/9(BusTBStartIn)
  NextBTIn/1 -> Backtracking_final/11(NextBTIn)
  P1_HW0/11(out_j) -> Backtracking_final/6(j)
  P1_HW0/3(EndMaxRAM (valor de i)) -> Backtracking_final/5(Maxi), delay_tc1/1
  Backtracking_final/1(BT_RAM_j(n)=i) -> _RAM_0/4(BT_RAM_j(n)=i)
  i(n-1)/1 -> Backtracking_final/10(i(n-1))
  Backtracking_final/4(BusMaxjOut) -> delay_tc7/1
  Backtracking_final/5(BusMaxiOut) -> delay_tc3/1
  BuxMaxiIn/1 -> Backtracking_final/8(BusMaxiIn)
  Backtracking_final/7(i(n)) -> delay_tc5/1
  Backtracking_final/2(BTRAMCont) -> _RAM_0/5(BTRAMCont)
  P1_HW0/4(EndMaxP (valor de j)) -> Backtracking_final/4(Maxj), delay_tc2/1
  P1_HW0/1(M_j(n)) -> M_j(n)/1
  P1_HW0/2(MaxValue) -> delay_tc/1
  P1_HW0/9(wEnd) -> _RAM_0/2(RAM_j(n)=i)
  P1_HW0/8(Direction) -> _RAM_0/3(D_j(n))
  P1_HW0/6(s(n-1)) -> s(n-1)/1
  P1_HW0/5(j) -> j+1/1
  P1_HW0/7(EnOut(n)) -> EnOut(n)/1
  seq_switch/2(q_j(n-1)) -> q_j(n)/1
  q_j(n)_/1 -> seq_switch/1(q_j(n))
  s_j(n)/1 -> P1_HW0/7(s(n))
  P1_HW0/10(TraceBackStart) -> Backtracking_final/3(TraceBackStart), Register1/1
  "reset "/1 -> P1_HW0/1("reset "), Backtracking_final/1("reset "), "delay_reset "/1, seq_switch/3("reset ")
  "delay_reset "/1 -> reset(n-1)/1
  Register10/1 -> "Out_DC "/1
  Register1/1 -> Traceback/1

== system SW_8/Subsystem/Subsystem3 ==
  "reset " : Inport
  M_j-1(n) : Inport  Port=2
  MaxValue_j-1 : Inport  Port=3
  EndMaxRAM_j-1 : Inport  Port=4
  EndMaxP_j-1 : Inport  Port=5
  j : Inport  Port=6
  EnIn(n) : Inport  Port=7
  q_j(n)_ : Inport  Port=8
  s_j(n) : Inport  Port=9
  BusMaxjIn : Inport  Port=10
  BuxMaxiIn : Inport  Port=11
  i(n-1) : Inport  Port=12
  BusTBStartIn : Inport  Port=13
  NextBTIn : Inport  Port=14
  Backtracking_final : Subsystem
  P1_HW0 : Subsystem
  Register1 : xbsIndex_r4/Register  init=0  rst=off  en=off  dbl_ovrd=off  block_type=register
  Register10 : xbsIndex_r4/Register  init=0  rst=off  en=off  dbl_ovrd=off  block_type=register
  _RAM_0 : Subsystem
  "delay_reset " : xbsIndex_r4/Register  init=0  rst=off  en=off  dbl_ovrd=off  block_type=register
  delay_tc{,1..7} (8 alike) : xbsIndex_r4/Register  init=0  rst=off  en=off  dbl_ovrd=off  block_type=register
  seq_switch : Subsystem
  "Out_DC " : Outport
  Traceback : Outport  Port=2
  reset(n-1) : Outport  Port=3
  M_j(n) : Outport  Port=4
  MaxValue : Outport  Port=5
  EndMaxRAM (valor de i) : Outport  Port=6
  EndMaxP (valor de j) : Outport  Port=7
  j+1 : Outport  Port=8
  EnOut(n) : Outport  Port=9
  q_j(n) : Outport  Port=10
  s(n-1) : Outport  Port=11
  BusMaxjOut : Outport  Port=12
  BusMaxiOut : Outport  Port=13
  i(n) : Outport  Port=14
  BusTBStartOut : Outport  Port=15
  NextBTOut : Outport  Port=16
  wires:
  Backtracking_final/3(Out_DC_j(n)) -> Register10/1
  _RAM_0/1(D_j(n)1) -> Backtracking_final/2("D(j)_n ")
  delay_tc7/1 -> BusMaxjOut/1
  delay_tc6/1 -> NextBTOut/1
  delay_tc5/1 -> i(n)/1
  delay_tc4/1 -> BusTBStartOut/1
  delay_tc3/1 -> BusMaxiOut/1
  delay_tc/1 -> MaxValue/1
  delay_tc2/1 -> EndMaxP (valor de j)/1
  delay_tc1/1 -> EndMaxRAM (valor de i)/1
  EndMaxRAM_j-1/1 -> P1_HW0/4(EndMaxRAM_j-1)
  M_j-1(n)/1 -> P1_HW0/2(M_j-1(n)1)
  j/1 -> P1_HW0/6(j-1)
  seq_switch/1(q_j) -> P1_HW0/9(q_j)
  MaxValue_j-1/1 -> P1_HW0/3(MaxValue_j-1)
  EndMaxP_j-1/1 -> P1_HW0/5(EndMaxP_j-1)
  EnIn(n)/1 -> P1_HW0/8(EnIn), seq_switch/2("Enable "), _RAM_0/1(En(n))
  Backtracking_final/6(BusTBStartOut) -> delay_tc4/1
  Backtracking_final/8(NextBTOut) -> delay_tc6/1
  BusMaxjIn/1 -> Backtracking_final/7(BusMaxjIn)
  BusTBStartIn/1 -> Backtracking_final/9(BusTBStartIn)
  NextBTIn/1 -> Backtracking_final/11(NextBTIn)
  P1_HW0/11(out_j) -> Backtracking_final/6(j)
  P1_HW0/3(EndMaxRAM (valor de i)) -> Backtracking_final/5(Maxi), delay_tc1/1
  Backtracking_final/1(BT_RAM_j(n)=i) -> _RAM_0/4(BT_RAM_j(n)=i)
  i(n-1)/1 -> Backtracking_final/10(i(n-1))
  Backtracking_final/4(BusMaxjOut) -> delay_tc7/1
  Backtracking_final/5(BusMaxiOut) -> delay_tc3/1
  BuxMaxiIn/1 -> Backtracking_final/8(BusMaxiIn)
  Backtracking_final/7(i(n)) -> delay_tc5/1
  Backtracking_final/2(BTRAMCont) -> _RAM_0/5(BTRAMCont)
  P1_HW0/4(EndMaxP (valor de j)) -> Backtracking_final/4(Maxj), delay_tc2/1
  P1_HW0/1(M_j(n)) -> M_j(n)/1
  P1_HW0/2(MaxValue) -> delay_tc/1
  P1_HW0/9(wEnd) -> _RAM_0/2(RAM_j(n)=i)
  P1_HW0/8(Direction) -> _RAM_0/3(D_j(n))
  P1_HW0/6(s(n-1)) -> s(n-1)/1
  P1_HW0/5(j) -> j+1/1
  P1_HW0/7(EnOut(n)) -> EnOut(n)/1
  seq_switch/2(q_j(n-1)) -> q_j(n)/1
  q_j(n)_/1 -> seq_switch/1(q_j(n))
  s_j(n)/1 -> P1_HW0/7(s(n))
  P1_HW0/10(TraceBackStart) -> Backtracking_final/3(TraceBackStart), Register1/1
  "reset "/1 -> P1_HW0/1("reset "), Backtracking_final/1("reset "), "delay_reset "/1, seq_switch/3("reset ")
  "delay_reset "/1 -> reset(n-1)/1
  Register10/1 -> "Out_DC "/1
  Register1/1 -> Traceback/1

== system SW_8/Subsystem/Subsystem4 ==
  "reset " : Inport
  M_j-1(n) : Inport  Port=2
  MaxValue_j-1 : Inport  Port=3
  EndMaxRAM_j-1 : Inport  Port=4
  EndMaxP_j-1 : Inport  Port=5
  j : Inport  Port=6
  EnIn(n) : Inport  Port=7
  q_j(n)_ : Inport  Port=8
  s_j(n) : Inport  Port=9
  BusMaxjIn : Inport  Port=10
  BuxMaxiIn : Inport  Port=11
  i(n-1) : Inport  Port=12
  BusTBStartIn : Inport  Port=13
  NextBTIn : Inport  Port=14
  Backtracking_final : Subsystem
  P1_HW0 : Subsystem
  Register1 : xbsIndex_r4/Register  init=0  rst=off  en=off  dbl_ovrd=off  block_type=register
  Register10 : xbsIndex_r4/Register  init=0  rst=off  en=off  dbl_ovrd=off  block_type=register
  _RAM_0 : Subsystem
  "delay_reset " : xbsIndex_r4/Register  init=0  rst=off  en=off  dbl_ovrd=off  block_type=register
  delay_tc{,1..7} (8 alike) : xbsIndex_r4/Register  init=0  rst=off  en=off  dbl_ovrd=off  block_type=register
  seq_switch : Subsystem
  "Out_DC " : Outport
  Traceback : Outport  Port=2
  reset(n-1) : Outport  Port=3
  M_j(n) : Outport  Port=4
  MaxValue : Outport  Port=5
  EndMaxRAM (valor de i) : Outport  Port=6
  EndMaxP (valor de j) : Outport  Port=7
  j+1 : Outport  Port=8
  EnOut(n) : Outport  Port=9
  q_j(n) : Outport  Port=10
  s(n-1) : Outport  Port=11
  BusMaxjOut : Outport  Port=12
  BusMaxiOut : Outport  Port=13
  i(n) : Outport  Port=14
  BusTBStartOut : Outport  Port=15
  NextBTOut : Outport  Port=16
  wires:
  Backtracking_final/3(Out_DC_j(n)) -> Register10/1
  _RAM_0/1(D_j(n)1) -> Backtracking_final/2("D(j)_n ")
  delay_tc7/1 -> BusMaxjOut/1
  delay_tc6/1 -> NextBTOut/1
  delay_tc5/1 -> i(n)/1
  delay_tc4/1 -> BusTBStartOut/1
  delay_tc3/1 -> BusMaxiOut/1
  delay_tc/1 -> MaxValue/1
  delay_tc2/1 -> EndMaxP (valor de j)/1
  delay_tc1/1 -> EndMaxRAM (valor de i)/1
  EndMaxRAM_j-1/1 -> P1_HW0/4(EndMaxRAM_j-1)
  M_j-1(n)/1 -> P1_HW0/2(M_j-1(n)1)
  j/1 -> P1_HW0/6(j-1)
  seq_switch/1(q_j) -> P1_HW0/9(q_j)
  MaxValue_j-1/1 -> P1_HW0/3(MaxValue_j-1)
  EndMaxP_j-1/1 -> P1_HW0/5(EndMaxP_j-1)
  EnIn(n)/1 -> P1_HW0/8(EnIn), seq_switch/2("Enable "), _RAM_0/1(En(n))
  Backtracking_final/6(BusTBStartOut) -> delay_tc4/1
  Backtracking_final/8(NextBTOut) -> delay_tc6/1
  BusMaxjIn/1 -> Backtracking_final/7(BusMaxjIn)
  BusTBStartIn/1 -> Backtracking_final/9(BusTBStartIn)
  NextBTIn/1 -> Backtracking_final/11(NextBTIn)
  P1_HW0/11(out_j) -> Backtracking_final/6(j)
  P1_HW0/3(EndMaxRAM (valor de i)) -> Backtracking_final/5(Maxi), delay_tc1/1
  Backtracking_final/1(BT_RAM_j(n)=i) -> _RAM_0/4(BT_RAM_j(n)=i)
  i(n-1)/1 -> Backtracking_final/10(i(n-1))
  Backtracking_final/4(BusMaxjOut) -> delay_tc7/1
  Backtracking_final/5(BusMaxiOut) -> delay_tc3/1
  BuxMaxiIn/1 -> Backtracking_final/8(BusMaxiIn)
  Backtracking_final/7(i(n)) -> delay_tc5/1
  Backtracking_final/2(BTRAMCont) -> _RAM_0/5(BTRAMCont)
  P1_HW0/4(EndMaxP (valor de j)) -> Backtracking_final/4(Maxj), delay_tc2/1
  P1_HW0/1(M_j(n)) -> M_j(n)/1
  P1_HW0/2(MaxValue) -> delay_tc/1
  P1_HW0/9(wEnd) -> _RAM_0/2(RAM_j(n)=i)
  P1_HW0/8(Direction) -> _RAM_0/3(D_j(n))
  P1_HW0/6(s(n-1)) -> s(n-1)/1
  P1_HW0/5(j) -> j+1/1
  P1_HW0/7(EnOut(n)) -> EnOut(n)/1
  seq_switch/2(q_j(n-1)) -> q_j(n)/1
  q_j(n)_/1 -> seq_switch/1(q_j(n))
  s_j(n)/1 -> P1_HW0/7(s(n))
  P1_HW0/10(TraceBackStart) -> Backtracking_final/3(TraceBackStart), Register1/1
  "reset "/1 -> P1_HW0/1("reset "), Backtracking_final/1("reset "), "delay_reset "/1, seq_switch/3("reset ")
  "delay_reset "/1 -> reset(n-1)/1
  Register10/1 -> "Out_DC "/1
  Register1/1 -> Traceback/1

== system SW_8/Subsystem/Subsystem5 ==
  "reset " : Inport
  M_j-1(n) : Inport  Port=2
  MaxValue_j-1 : Inport  Port=3
  EndMaxRAM_j-1 : Inport  Port=4
  EndMaxP_j-1 : Inport  Port=5
  j : Inport  Port=6
  EnIn(n) : Inport  Port=7
  q_j(n)_ : Inport  Port=8
  s_j(n) : Inport  Port=9
  BusMaxjIn : Inport  Port=10
  BuxMaxiIn : Inport  Port=11
  i(n-1) : Inport  Port=12
  BusTBStartIn : Inport  Port=13
  NextBTIn : Inport  Port=14
  Backtracking_final : Subsystem
  P1_HW0 : Subsystem
  Register1 : xbsIndex_r4/Register  init=0  rst=off  en=off  dbl_ovrd=off  block_type=register
  Register10 : xbsIndex_r4/Register  init=0  rst=off  en=off  dbl_ovrd=off  block_type=register
  _RAM_0 : Subsystem
  "delay_reset " : xbsIndex_r4/Register  init=0  rst=off  en=off  dbl_ovrd=off  block_type=register
  delay_tc{,1..7} (8 alike) : xbsIndex_r4/Register  init=0  rst=off  en=off  dbl_ovrd=off  block_type=register
  seq_switch : Subsystem
  "Out_DC " : Outport
  Traceback : Outport  Port=2
  reset(n-1) : Outport  Port=3
  M_j(n) : Outport  Port=4
  MaxValue : Outport  Port=5
  EndMaxRAM (valor de i) : Outport  Port=6
  EndMaxP (valor de j) : Outport  Port=7
  j+1 : Outport  Port=8
  EnOut(n) : Outport  Port=9
  q_j(n) : Outport  Port=10
  s(n-1) : Outport  Port=11
  BusMaxjOut : Outport  Port=12
  BusMaxiOut : Outport  Port=13
  i(n) : Outport  Port=14
  BusTBStartOut : Outport  Port=15
  NextBTOut : Outport  Port=16
  wires:
  Backtracking_final/3(Out_DC_j(n)) -> Register10/1
  _RAM_0/1(D_j(n)1) -> Backtracking_final/2("D(j)_n ")
  delay_tc7/1 -> BusMaxjOut/1
  delay_tc6/1 -> NextBTOut/1
  delay_tc5/1 -> i(n)/1
  delay_tc4/1 -> BusTBStartOut/1
  delay_tc3/1 -> BusMaxiOut/1
  delay_tc/1 -> MaxValue/1
  delay_tc2/1 -> EndMaxP (valor de j)/1
  delay_tc1/1 -> EndMaxRAM (valor de i)/1
  EndMaxRAM_j-1/1 -> P1_HW0/4(EndMaxRAM_j-1)
  M_j-1(n)/1 -> P1_HW0/2(M_j-1(n)1)
  j/1 -> P1_HW0/6(j-1)
  seq_switch/1(q_j) -> P1_HW0/9(q_j)
  MaxValue_j-1/1 -> P1_HW0/3(MaxValue_j-1)
  EndMaxP_j-1/1 -> P1_HW0/5(EndMaxP_j-1)
  EnIn(n)/1 -> P1_HW0/8(EnIn), seq_switch/2("Enable "), _RAM_0/1(En(n))
  Backtracking_final/6(BusTBStartOut) -> delay_tc4/1
  Backtracking_final/8(NextBTOut) -> delay_tc6/1
  BusMaxjIn/1 -> Backtracking_final/7(BusMaxjIn)
  BusTBStartIn/1 -> Backtracking_final/9(BusTBStartIn)
  NextBTIn/1 -> Backtracking_final/11(NextBTIn)
  P1_HW0/11(out_j) -> Backtracking_final/6(j)
  P1_HW0/3(EndMaxRAM (valor de i)) -> Backtracking_final/5(Maxi), delay_tc1/1
  Backtracking_final/1(BT_RAM_j(n)=i) -> _RAM_0/4(BT_RAM_j(n)=i)
  i(n-1)/1 -> Backtracking_final/10(i(n-1))
  Backtracking_final/4(BusMaxjOut) -> delay_tc7/1
  Backtracking_final/5(BusMaxiOut) -> delay_tc3/1
  BuxMaxiIn/1 -> Backtracking_final/8(BusMaxiIn)
  Backtracking_final/7(i(n)) -> delay_tc5/1
  Backtracking_final/2(BTRAMCont) -> _RAM_0/5(BTRAMCont)
  P1_HW0/4(EndMaxP (valor de j)) -> Backtracking_final/4(Maxj), delay_tc2/1
  P1_HW0/1(M_j(n)) -> M_j(n)/1
  P1_HW0/2(MaxValue) -> delay_tc/1
  P1_HW0/9(wEnd) -> _RAM_0/2(RAM_j(n)=i)
  P1_HW0/8(Direction) -> _RAM_0/3(D_j(n))
  P1_HW0/6(s(n-1)) -> s(n-1)/1
  P1_HW0/5(j) -> j+1/1
  P1_HW0/7(EnOut(n)) -> EnOut(n)/1
  seq_switch/2(q_j(n-1)) -> q_j(n)/1
  q_j(n)_/1 -> seq_switch/1(q_j(n))
  s_j(n)/1 -> P1_HW0/7(s(n))
  P1_HW0/10(TraceBackStart) -> Backtracking_final/3(TraceBackStart), Register1/1
  "reset "/1 -> P1_HW0/1("reset "), Backtracking_final/1("reset "), "delay_reset "/1, seq_switch/3("reset ")
  "delay_reset "/1 -> reset(n-1)/1
  Register10/1 -> "Out_DC "/1
  Register1/1 -> Traceback/1
